simulink model "PV_HP_HE_Tank_complete"  (R2018b)
settings: Solver=FixedStepAuto  StartTime=0.0  StopTime=24  FixedStep=1  RelTol=1e-3
values from neighbouring files (symbols this model uses):
  alpha_HE = 2500*3600    (= 9000000)    [Parameters_old MPC.m]
  beta_pv = 0.0045    [Parameters_old MPC.m]
  C_pair = 1006    [Parameters_old MPC.m]
  C_pw = 4182    [Parameters_old MPC.m]
  Cc = 11030    [Parameters_old MPC.m]
  Cev = 1897    [Parameters_old MPC.m]
  delta_HE = l_HE/4    (= 1)    [Parameters_old MPC.m]
  eta_pv = 0.15    [Parameters_old MPC.m]
  m_air = (2000 *1.225)    (= 2450)    [Parameters_old MPC.m]
  m_water = 10e-5*3600    (= 0.36)    [Parameters_old MPC.m]
  Npv = 6    [Parameters_old MPC.m]
  P_heater_max = 4000    [Parameters_old MPC.m]
  P_HP_max = 1000    [Parameters_old MPC.m]
  r_HE = 0.006    [Parameters_old MPC.m]
  rho_w = 1000    [Parameters_old MPC.m]
  T_HE_0 = 273+40    (= 313)    [Parameters_old MPC.m]
  T_NOCT = 45    [Parameters_old MPC.m]
  T_ref = 25    [Parameters_old MPC.m]
  T_tank_0 = 273+15    (= 288)    [Parameters_old MPC.m]
  V_t = 0.3    [Parameters_old MPC.m]
settings Model: Creator=enzlp  LastModifiedBy=enzlp

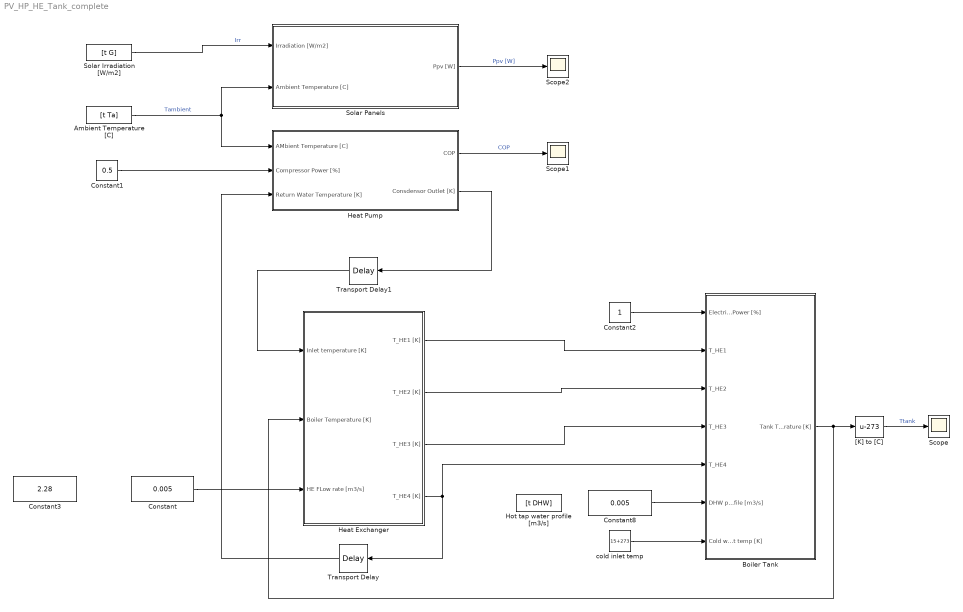
== system PV_HP_HE_Tank_complete ==
  Ambient Temperature [C] : FromWorkspace  VariableName=[t Ta]  SampleTime=0
  Boiler Tank : Subsystem
  Constant : Constant  Value=0.005
  Constant1 : Constant  Value=0.5
  Constant2 : Constant
  Constant3 : Constant  Value=2.28
  Constant8 : Constant  Value=0.005
  Heat Exchanger : Subsystem
  Heat Pump : Subsystem
  Hot tap water profile [m3/s] : FromWorkspace  VariableName=[t DHW]  SampleTime=0
  Scope : Scope
  Scope1 : Scope
  Scope2 : Scope
  Solar Irradiation [W/m2] : FromWorkspace  VariableName=[t G]  SampleTime=0
  Solar Panels : Subsystem
  Transport Delay : TransportDelay  InitialOutput=10+273
  Transport Delay1 : TransportDelay  InitialOutput=10+273
  "[K] to [C]" : Bias  Bias=-273
  cold inlet temp : Constant  Value=15+273
  wires:
  Ambient Temperature [C]/1 -> Heat Pump/1(AMbient Temperature [C]), Solar Panels/2(Ambient Temperature [C])  "Tambient"
  Heat Pump/1(COP) -> Scope1/1  "COP"
  cold inlet temp/1 -> Boiler Tank/7(Cold water inlet temp [K])
  "[K] to [C]"/1 -> Scope/1  "Ttank"
  Solar Panels/1(Ppv [W]) -> Scope2/1  "Ppv [W]"
  Constant8/1 -> Boiler Tank/6(DHW profile [m3/s])
  Solar Irradiation [W/m2]/1 -> Solar Panels/1(Irradiation [W/m2])  "Irr"
  Constant/1 -> Heat Exchanger/3(HE FLow rate [m3/s])
  Constant1/1 -> Heat Pump/2(Compressor Power [%])
  Constant2/1 -> Boiler Tank/1(Electric Power [%])
  Heat Exchanger/4(T_HE4 [K]) -> Transport Delay/1, Boiler Tank/5(T_HE4)
  Heat Pump/2(Consdensor Outlet [K]) -> Transport Delay1/1
  Transport Delay/1 -> Heat Pump/3(Return Water Temperature [K])
  Boiler Tank/1(Tank Temperature [K]) -> Heat Exchanger/2(Boiler Temperature [K]), "[K] to [C]"/1
  Transport Delay1/1 -> Heat Exchanger/1(Inlet temperature [K])
  Heat Exchanger/1(T_HE1 [K]) -> Boiler Tank/2(T_HE1)
  Heat Exchanger/2(T_HE2 [K]) -> Boiler Tank/3(T_HE2)
  Heat Exchanger/3(T_HE3 [K]) -> Boiler Tank/4(T_HE3)

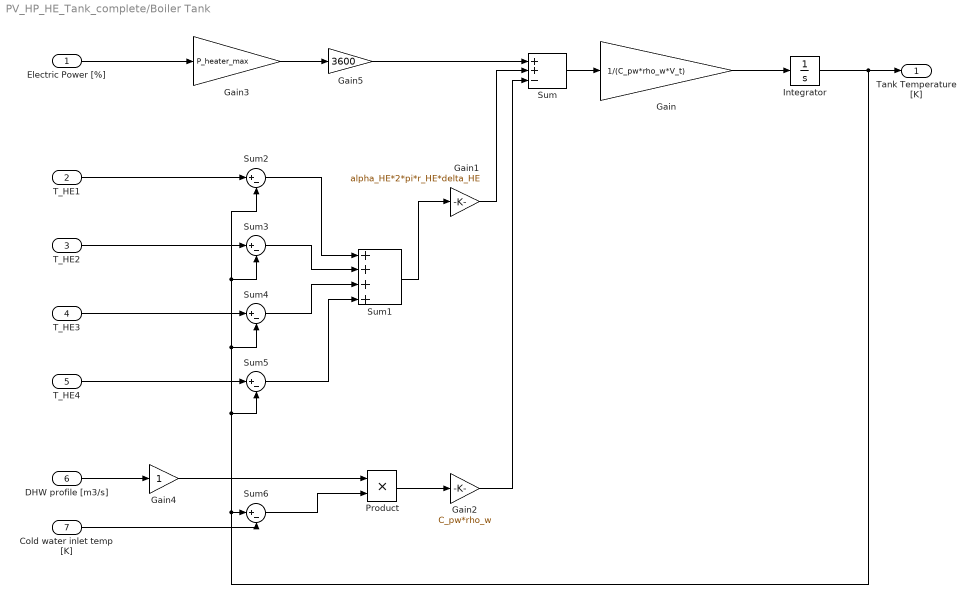
== system PV_HP_HE_Tank_complete/Boiler Tank ==
  Electric Power [%] : Inport
  T_HE1 : Inport  Port=2
  T_HE2 : Inport  Port=3
  T_HE3 : Inport  Port=4
  T_HE4 : Inport  Port=5
  DHW profile [m3/s] : Inport  Port=6
  Cold water inlet temp [K] : Inport  Port=7
  Gain : Gain  Gain=1/(C_pw*rho_w*V_t)
  Gain1 : Gain  Gain=alpha_HE*2*pi*r_HE*delta_HE
  Gain2 : Gain  Gain=C_pw*rho_w
  Gain3 : Gain  Gain=P_heater_max
  Gain4 : Gain
  Gain5 : Gain  Gain=3600
  Integrator : Integrator  InitialCondition=T_tank_0
  Product : Product
  Sum : Sum  Inputs=++-
  Sum1 : Sum  Inputs=++++
  Sum{2..6} (5 alike) : Sum  Inputs=|+-
  Tank Temperature [K] : Outport
  wires:
  Cold water inlet temp [K]/1 -> Sum6/2
  Product/1 -> Gain2/1
  Integrator/1 -> Sum2/2, Sum3/2, Sum4/2, Sum5/2, Sum6/1, Tank Temperature [K]/1
  Sum5/1 -> Sum1/4
  T_HE4/1 -> Sum5/1
  Sum4/1 -> Sum1/3
  Sum/1 -> Gain/1
  Gain/1 -> Integrator/1
  Gain1/1 -> Sum/2
  Gain2/1 -> Sum/3
  Sum6/1 -> Product/2
  Gain4/1 -> Product/1
  Sum2/1 -> Sum1/1
  Sum1/1 -> Gain1/1
  Sum3/1 -> Sum1/2
  Gain3/1 -> Gain5/1
  T_HE1/1 -> Sum2/1
  T_HE2/1 -> Sum3/1
  T_HE3/1 -> Sum4/1
  Electric Power [%]/1 -> Gain3/1
  DHW profile [m3/s]/1 -> Gain4/1
  Gain5/1 -> Sum/1

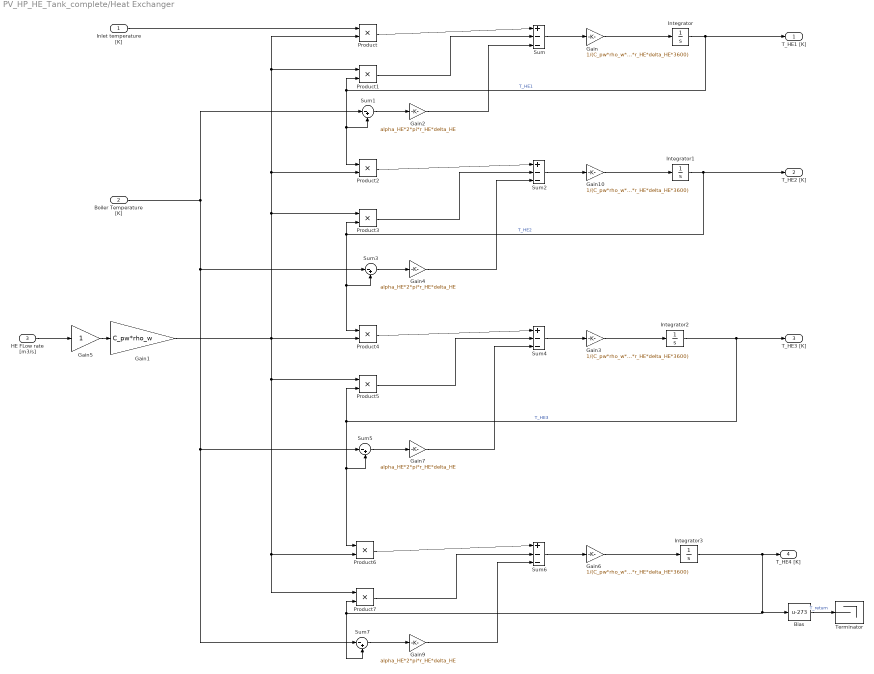
== system PV_HP_HE_Tank_complete/Heat Exchanger ==
  Inlet temperature [K] : Inport
  Boiler Temperature [K] : Inport  Port=2
  HE FLow rate [m3/s] : Inport  Port=3
  Bias : Bias  Bias=-273
  Gain{,3,6,10} (4 alike) : Gain  Gain=1/(C_pw*rho_w*pi*r_HE*r_HE*delta_HE*3600)
  Gain1 : Gain  Gain=C_pw*rho_w
  Gain{2,4,7,9} (4 alike) : Gain  Gain=alpha_HE*2*pi*r_HE*delta_HE
  Gain5 : Gain
  Integrator{,1..3} (4 alike) : Integrator  InitialCondition=T_HE_0
  Product{,1..7} (8 alike) : Product
  Sum{,2,4,6} (4 alike) : Sum  Inputs=|+--
  Sum{1,3,5,7} (4 alike) : Sum  Inputs=|-+
  Terminator : Terminator
  T_HE1 [K] : Outport
  T_HE2 [K] : Outport  Port=2
  T_HE3 [K] : Outport  Port=3
  T_HE4 [K] : Outport  Port=4
  wires:
  Bias/1 -> Terminator/1  "T_return"
  HE FLow rate [m3/s]/1 -> Gain5/1
  Gain/1 -> Integrator/1
  Sum/1 -> Gain/1
  Product/1 -> Sum/1
  Gain5/1 -> Gain1/1
  Inlet temperature [K]/1 -> Product/1
  Gain1/1 -> Product7/1, Product6/2, Product5/1, Product3/1, Product2/2, Product1/1, Product/2, Product4/2
  Integrator/1 -> T_HE1 [K]/1, Product1/2, Product2/1, Sum1/2  "T_HE1"
  Product1/1 -> Sum/2
  Boiler Temperature [K]/1 -> Sum7/1, Sum5/1, Sum3/1, Sum1/1
  Sum1/1 -> Gain2/1
  Gain2/1 -> Sum/3
  Gain10/1 -> Integrator1/1
  Product2/1 -> Sum2/1
  Integrator1/1 -> T_HE2 [K]/1, Product3/2, Sum3/2, Product4/1  "T_HE2"
  Sum2/1 -> Gain10/1
  Product3/1 -> Sum2/2
  Sum3/1 -> Gain4/1
  Gain4/1 -> Sum2/3
  Integrator2/1 -> Product5/2, Product6/1, Sum5/2, T_HE3 [K]/1  "T_HE3"
  Gain3/1 -> Integrator2/1
  Sum4/1 -> Gain3/1
  Product4/1 -> Sum4/1
  Product5/1 -> Sum4/2
  Sum5/1 -> Gain7/1
  Gain7/1 -> Sum4/3
  Integrator3/1 -> Product7/2, Sum7/2, Bias/1, T_HE4 [K]/1
  Gain6/1 -> Integrator3/1
  Sum6/1 -> Gain6/1
  Product6/1 -> Sum6/1
  Product7/1 -> Sum6/2
  Sum7/1 -> Gain9/1
  Gain9/1 -> Sum6/3

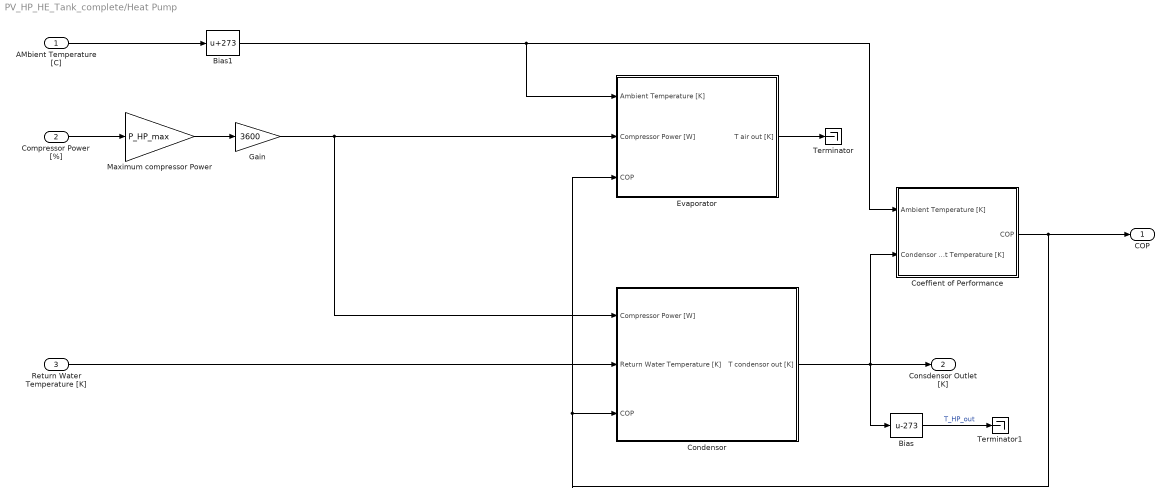
== system PV_HP_HE_Tank_complete/Heat Pump ==
  AMbient Temperature [C] : Inport
  Compressor Power [%] : Inport  Port=2
  Return Water Temperature [K] : Inport  Port=3
  Bias : Bias  Bias=-273
  Bias1 : Bias  Bias=273
  Coeffient of Performance : Subsystem
  Condensor : Subsystem
  Evaporator : Subsystem
  Gain : Gain  Gain=3600
  Maximum compressor Power : Gain  Gain=P_HP_max
  Terminator : Terminator
  Terminator1 : Terminator
  COP : Outport
  Consdensor Outlet [K] : Outport  Port=2
  wires:
  Bias1/1 -> Evaporator/1(Ambient Temperature [K]), Coeffient of Performance/1(Ambient Temperature [K])
  Compressor Power [%]/1 -> Maximum compressor Power/1
  Maximum compressor Power/1 -> Gain/1
  Evaporator/1(T air out [K]) -> Terminator/1
  Return Water Temperature [K]/1 -> Condensor/2(Return Water Temperature [K])
  AMbient Temperature [C]/1 -> Bias1/1
  Condensor/1(T condensor out [K]) -> Bias/1, Consdensor Outlet [K]/1, Coeffient of Performance/2(Condensor outet Temperature [K])
  Bias/1 -> Terminator1/1  "T_HP_out"
  Coeffient of Performance/1(COP) -> Condensor/3(COP), Evaporator/3(COP), COP/1
  Gain/1 -> Condensor/1(Compressor Power [W]), Evaporator/2(Compressor Power [W])

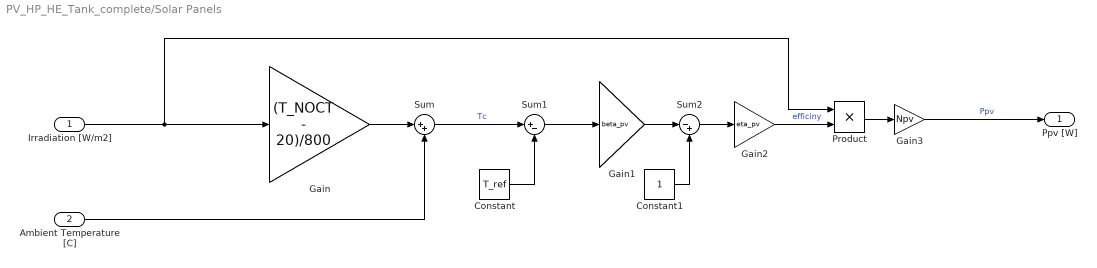
== system PV_HP_HE_Tank_complete/Solar Panels ==
  Irradiation [W/m2] : Inport
  Ambient Temperature [C] : Inport  Port=2
  Constant : Constant  Value=T_ref
  Constant1 : Constant
  Gain : Gain  Gain=(T_NOCT - 20)/800
  Gain1 : Gain  Gain=beta_pv
  Gain2 : Gain  Gain=eta_pv
  Gain3 : Gain  Gain=Npv
  Product : Product
  Sum : Sum  Inputs=|++
  Sum1 : Sum  Inputs=|+-
  Sum2 : Sum  Inputs=|-+
  Ppv [W] : Outport
  wires:
  Gain3/1 -> Ppv [W]/1  "Ppv"
  Sum1/1 -> Gain1/1
  Gain/1 -> Sum/1
  Constant1/1 -> Sum2/2
  Sum/1 -> Sum1/1  "Tc"
  Sum2/1 -> Gain2/1
  Constant/1 -> Sum1/2
  Gain2/1 -> Product/2  "efficiny"
  Gain1/1 -> Sum2/1
  Irradiation [W/m2]/1 -> Product/1, Gain/1
  Product/1 -> Gain3/1
  Ambient Temperature [C]/1 -> Sum/2

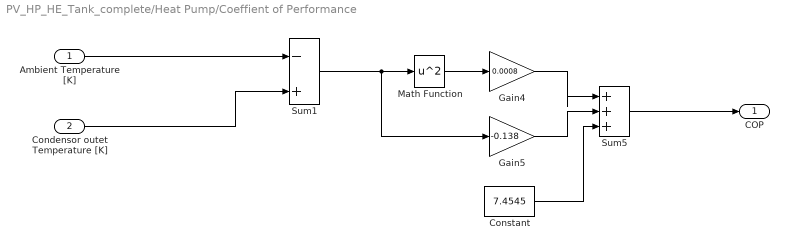
== system PV_HP_HE_Tank_complete/Heat Pump/Coeffient of Performance ==
  Ambient Temperature [K] : Inport
  Condensor outet Temperature [K] : Inport  Port=2
  Constant : Constant  Value=7.4545
  Gain4 : Gain  Gain=0.0008
  Gain5 : Gain  Gain=-0.138
  Math Function : Math  Operator=square  SaturateOnIntegerOverflow=on
  Sum1 : Sum  Inputs=|-+
  Sum5 : Sum  Inputs=|+++
  COP : Outport
  wires:
  Sum1/1 -> Gain5/1, Math Function/1
  Condensor outet Temperature [K]/1 -> Sum1/2
  Gain4/1 -> Sum5/1
  Constant/1 -> Sum5/3
  Gain5/1 -> Sum5/2
  Sum5/1 -> COP/1
  Ambient Temperature [K]/1 -> Sum1/1
  Math Function/1 -> Gain4/1

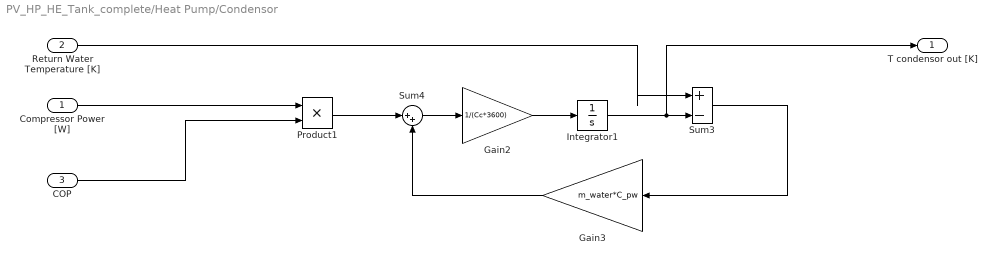
== system PV_HP_HE_Tank_complete/Heat Pump/Condensor ==
  Compressor Power [W] : Inport
  Return Water Temperature [K] : Inport  Port=2
  COP : Inport  Port=3
  Gain2 : Gain  Gain=1/(Cc*3600)
  Gain3 : Gain  Gain=m_water*C_pw
  Integrator1 : Integrator  InitialCondition=10+273
  Product1 : Product
  Sum3 : Sum  Inputs=|+-
  Sum4 : Sum  Inputs=|++
  T condensor out [K] : Outport
  wires:
  Gain3/1 -> Sum4/2
  Sum4/1 -> Gain2/1
  Integrator1/1 -> T condensor out [K]/1, Sum3/2
  Compressor Power [W]/1 -> Product1/1
  Return Water Temperature [K]/1 -> Sum3/1
  Gain2/1 -> Integrator1/1
  Sum3/1 -> Gain3/1
  Product1/1 -> Sum4/1
  COP/1 -> Product1/2

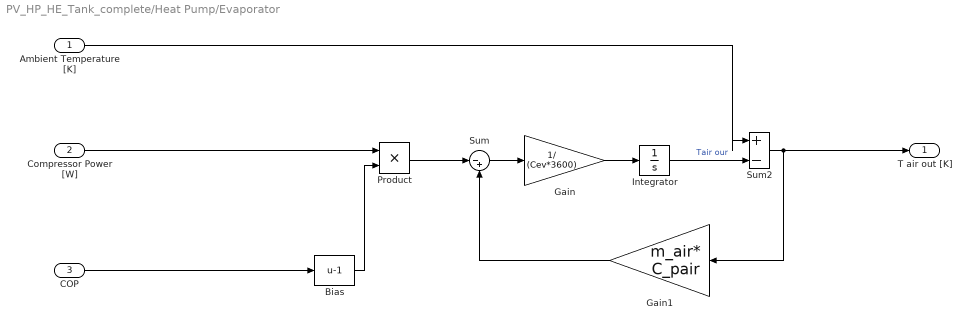
== system PV_HP_HE_Tank_complete/Heat Pump/Evaporator ==
  Ambient Temperature [K] : Inport
  Compressor Power [W] : Inport  Port=2
  COP : Inport  Port=3
  Bias : Bias  Bias=-1
  Gain : Gain  Gain=1/ (Cev*3600)
  Gain1 : Gain  Gain=m_air* C_pair
  Integrator : Integrator  InitialCondition=10
  Product : Product
  Sum : Sum  Inputs=|-+
  Sum2 : Sum  Inputs=|+-
  T air out [K] : Outport
  wires:
  Compressor Power [W]/1 -> Product/1
  Sum/1 -> Gain/1
  Gain1/1 -> Sum/2
  Integrator/1 -> Sum2/2  "Tair our"
  Sum2/1 -> T air out [K]/1, Gain1/1
  Gain/1 -> Integrator/1
  Ambient Temperature [K]/1 -> Sum2/1
  Bias/1 -> Product/2
  Product/1 -> Sum/1
  COP/1 -> Bias/1
